simulink model "BPF_Acivity2"  (R2022a)
settings: Solver=VariableStepAuto  StartTime=0.0  StopTime=10.0  RelTol=1e-3
values from neighbouring files (symbols this model uses):
  Vary_Sine_Feq = Vary_Sine_Var    [Run_Sim_BPF.m]
libraries: dsparch4 x2, dspsrcs4 x1
settings Model: Creator=chadw  LastModifiedBy=chadw

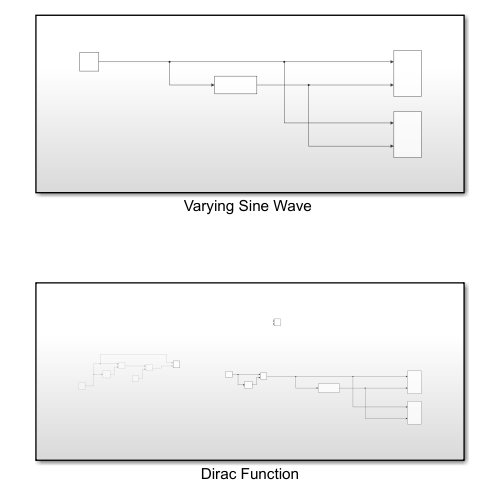
[thumbnail: Simulink's stored preview of the top-level diagram]
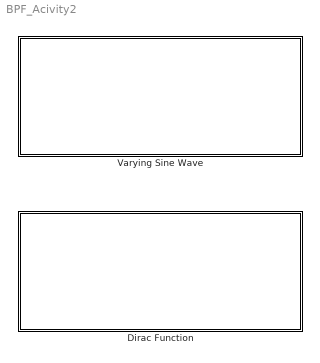
== system BPF_Acivity2 ==
  Dirac Function : Subsystem
  "Varying Sine Wave " : Subsystem

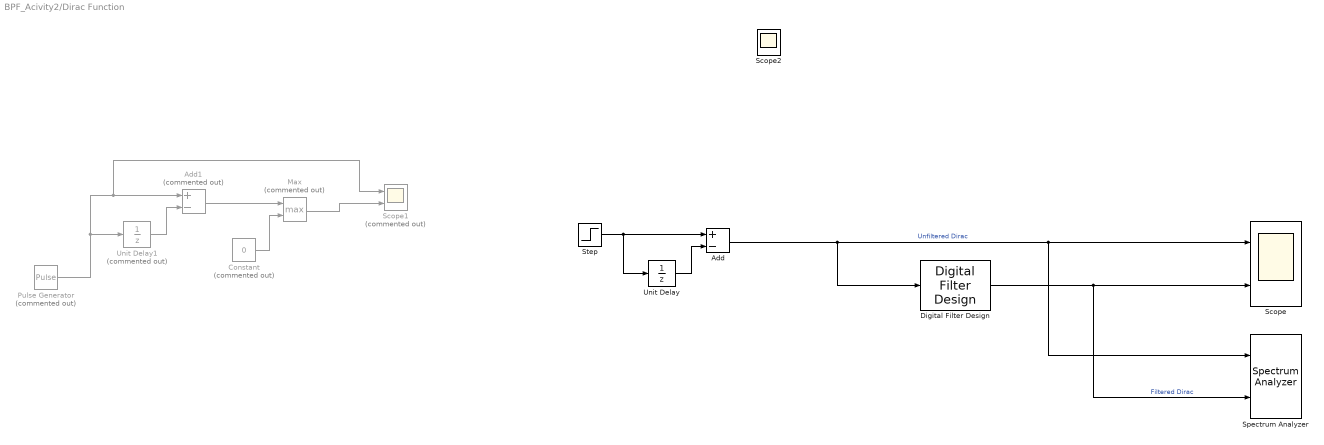
== system BPF_Acivity2/Dirac Function ==
  Add : Sum  Inputs=+-
  Add1 : Sum  Commented=on  Inputs=+-
  Constant : Constant  Commented=on  Value=0
  Digital Filter Design : dsparch4/Digital Filter Design  mwdsp_browser_bugfix_var=off
  Max : MinMax  Commented=on  Function=max  Inputs=2
  Pulse Generator : DiscretePulseGenerator  Commented=on  PulseType=Time based  Period=10  PulseWidth=5  PhaseDelay=2
  Scope : Scope  NumInputPorts=2
  Scope1 : Scope  Commented=on  NumInputPorts=2
  Scope2 : Scope  NumInputPorts=2
  Spectrum Analyzer : SpectrumAnalyzer  NumInputPorts=2
  Step : Step  SampleTime=1/1000
  Unit Delay : UnitDelay  SampleTime=-1  HasFrameUpgradeWarning=on
  Unit Delay1 : UnitDelay  Commented=on  SampleTime=-1  HasFrameUpgradeWarning=on
  wires:
  Add/1 -> Digital Filter Design/1, Spectrum Analyzer/1, Scope/1  "Unfiltered Dirac"
  Digital Filter Design/1 -> Spectrum Analyzer/2, Scope/2  "Filtered Dirac"
  Step/1 -> Unit Delay/1, Add/1
  Unit Delay/1 -> Add/2
  Unit Delay1/1 -> Add1/2
  Add1/1 -> Max/1
  Pulse Generator/1 -> Unit Delay1/1, Scope1/1, Add1/1
  Max/1 -> Scope1/2
  Constant/1 -> Max/2

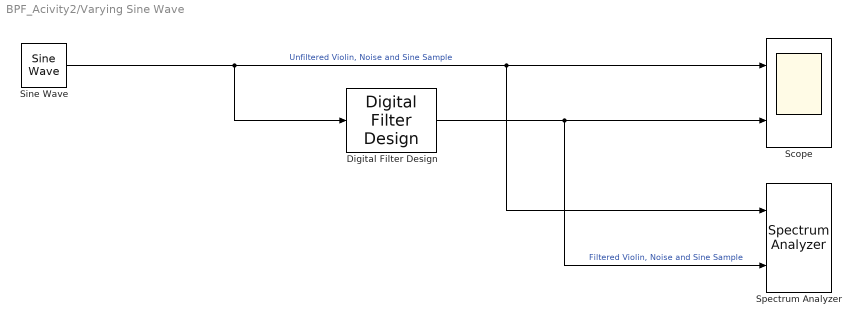
== system BPF_Acivity2/Varying Sine Wave  ==
  Digital Filter Design : dsparch4/Digital Filter Design  mwdsp_browser_bugfix_var=off
  Scope : Scope  NumInputPorts=2
  Sine Wave : dspsrcs4/Sine Wave  Amplitude=1  Frequency=Vary_Sine_Feq  Phase=0  SampleMode=Discrete  OutComplex=Real  CompMethod=Trigonometric fcn  TableSize=Speed  SampleTime=1/1000  SamplesPerFrame=1  ResetState=Restart at time zero  OutputFrames=off  dataType=double  wordLen=16  udDataType=sfix(16)  fracBitsMode=Best precision  numFracBits=15  OutDataTypeStr=double  LastOutDataTypeStr=double
  Spectrum Analyzer : SpectrumAnalyzer  NumInputPorts=2
  wires:
  Digital Filter Design/1 -> Scope/2, Spectrum Analyzer/2  "Filtered Violin, Noise and Sine Sample"
  Sine Wave/1 -> Digital Filter Design/1, Scope/1, Spectrum Analyzer/1  "Unfiltered Violin, Noise and Sine Sample"
